simulink library "M_MK"  (R2025a)
settings: Solver=VariableStepAuto  StartTime=0.0  StopTime=10.0  RelTol=1e-3
settings Model: Creator=Szalay  LastModifiedBy=Szalay

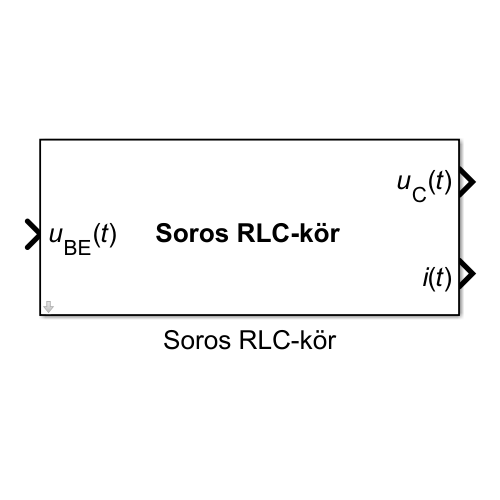
[thumbnail: Simulink's stored preview of the top-level diagram]
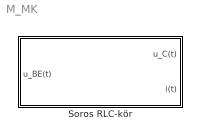
== system M_MK ==
  Soros RLC-kör : Subsystem  mask(Soros RLC-kör){L=1e-3, R=1, tau=1e-6, u_C0=0, i_0=0}
      mask prompts: L "Öninduktivitás (H)"; R "Ellenállás (Ohm)"; tau "Időállandó"; u_C0 "A kapacitáson eső feszültség kezdeti értéke (V)"; i_0 "Kezdeti áramerősség (A)"
      mask help: A soros RLC-kör modellje.
      mask DialogControl ParameterGroupVar Prompt: Az ismert jellemzők
      mask DialogControl Container3 Prompt: Kezdeti értékek
      mask Display:
      | % Csatlakozók
      | port_label('input', 1, '{\itu}_{BE}({\itt})', 'texmode', 'on');
      | port_label('output', 1, '{\itu}_{C}({\itt})', 'texmode', 'on');
      | port_label('output', 2, '{\iti}({\itt})', 'texmode', 'on');
      | 
      | % Felirat
      | text(0.5, 0.5, '{\bfSoros RLC-kör}', ...
      |     'HorizontalAlignment', 'center', 'Interpreter', 'tex' ...
      | );

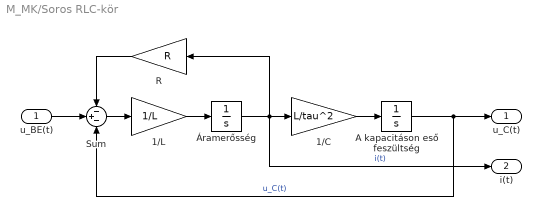
== system M_MK/Soros RLC-kör ==
  u_BE(t) : Inport
  1/C : Gain  Gain=L/tau^2
  1/L : Gain  Gain=1/L
  A kapacitáson eső feszültség : Integrator  InitialCondition=u_C0
  R : Gain  Gain=R
  Sum : Sum  Inputs=-+-
  Áramerősség : Integrator  InitialCondition=i_0
  u_C(t) : Outport
  i(t) : Outport  Port=2
  wires:
  Sum/1 -> 1/L/1
  u_BE(t)/1 -> Sum/2
  R/1 -> Sum/1
  Áramerősség/1 -> 1/C/1, i(t)/1, R/1  "i(t)"
  A kapacitáson eső feszültség/1 -> u_C(t)/1, Sum/3  "u_C(t)"
  1/L/1 -> Áramerősség/1
  1/C/1 -> A kapacitáson eső feszültség/1
